simulink model "relation_operator_4"  (R2021a)
settings: Solver=VariableStepAuto  StartTime=0.0  StopTime=10.0  MaxStep=1e-3  RelTol=1e-3
libraries: simulink x2
settings Model: Creator=yasso  LastModifiedBy=yasso

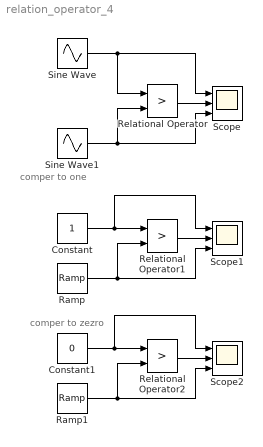
== system relation_operator_4 ==
  note: comper to zezro
  note: comper to one
  Constant : Constant
  Constant1 : Constant  Value=0
  Ramp : simulink/Sources/Ramp  slope=1  start=0  InitialOutput=-2
  Ramp1 : simulink/Sources/Ramp  slope=1  start=0  InitialOutput=-2
  Relational Operator : RelationalOperator  Operator=>  OutDataTypeStr=boolean  RndMeth=Simplest
  Relational Operator1 : RelationalOperator  Operator=>  OutDataTypeStr=boolean  RndMeth=Simplest
  Relational Operator2 : RelationalOperator  Operator=>  OutDataTypeStr=boolean  RndMeth=Simplest
  Scope : Scope  NumInputPorts=3
  Scope1 : Scope  NumInputPorts=3
  Scope2 : Scope  NumInputPorts=3
  Sine Wave : Sin  SampleTime=0
  Sine Wave1 : Sin  Phase=-pi  SampleTime=0
  wires:
  Sine Wave/1 -> Scope/1, Relational Operator/1
  Sine Wave1/1 -> Scope/3, Relational Operator/2
  Relational Operator/1 -> Scope/2
  Relational Operator1/1 -> Scope1/2
  Ramp/1 -> Relational Operator1/2, Scope1/3
  Constant/1 -> Scope1/1, Relational Operator1/1
  Constant1/1 -> Relational Operator2/1, Scope2/1
  Ramp1/1 -> Scope2/3, Relational Operator2/2
  Relational Operator2/1 -> Scope2/2
